simulink model "EnabledSubsystem"  (R2015b)
settings: Solver=VariableStepAuto  StartTime=0.0  StopTime=10.0  MaxStep=0.01  RelTol=1e-3
settings Model: Creator=LUBO  LastModifiedBy=LUBO

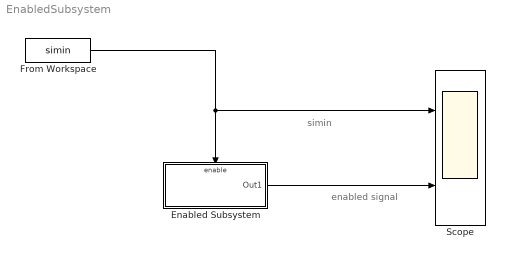
== system EnabledSubsystem ==
  note: simin
  note: enabled signal
  Enabled Subsystem : Subsystem  TreatAsAtomicUnit=on
  From Workspace : FromWorkspace  VariableName=simin  SampleTime=0
  Scope : Scope  NumInputPorts=2
  wires:
  From Workspace/1 -> Enabled Subsystem/Enable, Scope/1
  Enabled Subsystem/1(Out1) -> Scope/2

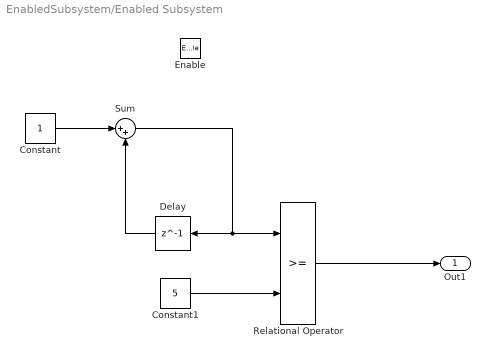
== system EnabledSubsystem/Enabled Subsystem ==
  Enable : EnablePort  StatesWhenEnabling=reset
  Constant : Constant
  Constant1 : Constant  Value=5
  Delay : Delay  DelayLength=1  InitialCondition=0  SampleTime=1
  Relational Operator : RelationalOperator  OutDataTypeStr=boolean
  Sum : Sum  Inputs=|++
  Out1 : Outport
  wires:
  Relational Operator/1 -> Out1/1
  Constant1/1 -> Relational Operator/2
  Constant/1 -> Sum/1
  Sum/1 -> Delay/1, Relational Operator/1
  Delay/1 -> Sum/2
